simulink model "Boat_Response"  (R2022b)
settings: Solver=VariableStepAuto  StartTime=0.0  StopTime=20  RelTol=0.1
model workspace (MAT data in the model file):
  Air_Kinematic_Viscosity = 1.48e-05
  Air_density = 1.225
  Angle_Breakpoints = [-10.5 -10.25 -10 -9.75 -9.5 -9.25 -9 -8.75 -8.5 -8.25 -8 -7.75 -7.5 -7.25 -7 -6.75 -6.5 -6.25 -6 -5.75 -5.5 -5.25 -5 -4.75 -4.5 -4.25 -4 -3.75 -3.5 -3.25 -3 -2.75 -2.5 -2.25 -2 -1.75 -1.5 -1.25 -1 -0.75 -0.5 -0.25 0 0.25 0.5 0.75 1 1.25 1.5 1.75 2 2.25 2.5 2.75 3 3.25 3.5 3.75 4 4.25 4.5 4.75 5 5.25 5.5 5.75 6 6.25 6.5 6.75 7 7.25 7.5 7.75 8 8.25 8.5 8.75 9 9.25 9.5 9.75 10 10.25 10.5]
  Boat_Slosh_Damping = 1500
  Keel_Area = 1
  Keel_Bulb_COG = 1.3
  Keel_Bulb_Mass = 70
  Keel_Chord = 0.7
  Keel_Fin_COG = 0.8
  Keel_Fin_COP = 0.7
  Keel_Fin_Mass = 8
  M_per_s_to_knots = 1.944
  NACA_0018_Drag_LU = [0.10841 0.10247 0.08947 0.06466 0.05594 0.05095 0.05074 0.04743 0.04673 0.04411 0.04386 0.04172 ... (425 elements, 85x5)]
  NACA_0018_Lift_LU = [-0.4876 -0.5001 -0.5715 -0.7409 -0.8387 -0.8938 -0.8627 -0.8928 -0.8721 -0.8918 -0.8647 -0.8747 ... (425 elements, 85x5)]
  Resistance_Curve = [0; 0.03; 0.11; 0.23; 0.39; 0.58; 0.85; 1.14; 1.49; 1.88; 2.53; 2.87; 3.31; 4.43; 6.4; 6.73; 6.99; 7.38; 13.49; 23.01; 22.15; 20.72; 36.03; 62.97; 86.69; 98.27; 97.94; 90.93; 82.95; 77.95; 77.69; 82.27; 90.87; 102.29; 115.35; 129.07; 142.7; 155.72; 167.84; 178.9; 188.84]
  Resistance_Curve_Velocity_BreakPoints = [0; 0.125; 0.25; 0.375; 0.5; 0.625; 0.75; 0.875; 1; 1.125; 1.25; 1.375; 1.5; 1.625; 1.75; 1.875; 2; 2.125; 2.25; 2.375; 2.5; 2.625; 2.75; 2.875; 3; 3.125; 3.25; 3.375; 3.5; 3.625; 3.75; 3.875; 4; 4.125; 4.25; 4.375; 4.5; 4.625; 4.75; 4.875; 5]
  Reynolds_Breakpoints = [50000 100000 200000 500000 1000000]
  Sail_Area = 2
  Sail_Best_Angles = [5.75 6.75 7 9.25 10]
  Sail_COG = 1.35
  Sail_COP = 1.5
  Sail_Chord = 1.3
  Sail_Mass = 32
  Sig = Simulink.Signal
  Sig.DataType = 'auto'
  Sig.Dimensions = -1
  Sig.DimensionsMode = 'auto'
  Sig.Complexity = 'auto'
  Sig.SampleTime = -1
  Sig.SamplingMode = 'auto'
  Total_MMOI = 200
  Total_Mass = 250
  Water_Density = 997
  Water_Kinematic_Viscosity = 1.3e-06
libraries: simulink_extras x13, vrlib x1, SignalEditorBlockLib x1
settings Model: Creator=ewanb  LastModifiedBy=ewanb
settings SolverCC: ZeroCrossAlgorithm=Adaptive
settings DebuggingCC: IgnoredZcDiagnostic=none

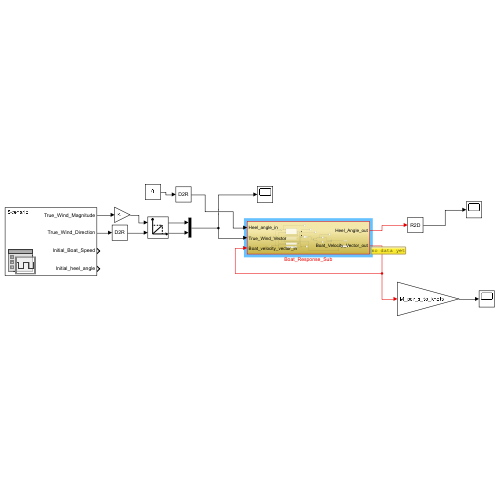
[thumbnail: Simulink's stored preview of the top-level diagram]
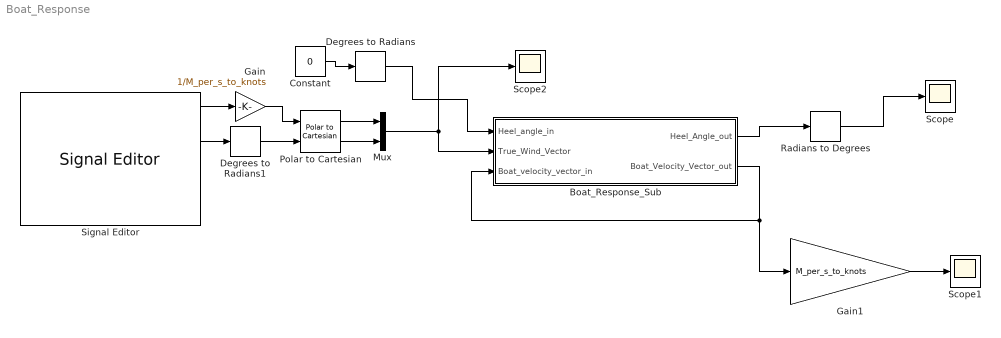
== system Boat_Response ==
  Boat_Response_Sub : Subsystem
  Constant : Constant  Value=0
  Degrees to Radians : simulink_extras/Transformations/Degrees to Radians
  Degrees to Radians1 : simulink_extras/Transformations/Degrees to Radians
  Gain : Gain  Gain=1/M_per_s_to_knots
  Gain1 : Gain  Gain=M_per_s_to_knots
  Mux : Mux  Inputs=2
  Polar to Cartesian : simulink_extras/Transformations/Polar to Cartesian
  Radians to Degrees : simulink_extras/Transformations/Radians to Degrees
  Scope : Scope
  Scope1 : Scope
  Scope2 : Scope
  Signal Editor : SignalEditorBlockLib/Signal Editor  FileName=10knts_Beam_Reach.mat  ActiveScenario=Scenario  ActiveSignal=True_Wind_Magnitude  IsBus=off  OutputBusObjectStr=Bus: BusObject  SampleTime=0  Interpolate=off  ZeroCross=off  OutputAfterFinalValue=Setting to zero  Unit=inherit  PreserveSignalName=on
  wires:
  Polar to Cartesian/1 -> Mux/1
  Mux/1 -> Boat_Response_Sub/2(True_Wind_Vector), Scope2/1
  Polar to Cartesian/2 -> Mux/2
  Radians to Degrees/1 -> Scope/1
  Boat_Response_Sub/1(Heel_Angle_out) -> Radians to Degrees/1
  Boat_Response_Sub/2(Boat_Velocity_Vector_out) -> Gain1/1, Boat_Response_Sub/3(Boat_velocity_vector_in)
  Degrees to Radians1/1 -> Polar to Cartesian/2
  Signal Editor/2 -> Degrees to Radians1/1
  Degrees to Radians/1 -> Boat_Response_Sub/1(Heel_angle_in)
  Constant/1 -> Degrees to Radians/1
  Gain/1 -> Polar to Cartesian/1
  Signal Editor/1 -> Gain/1
  Gain1/1 -> Scope1/1

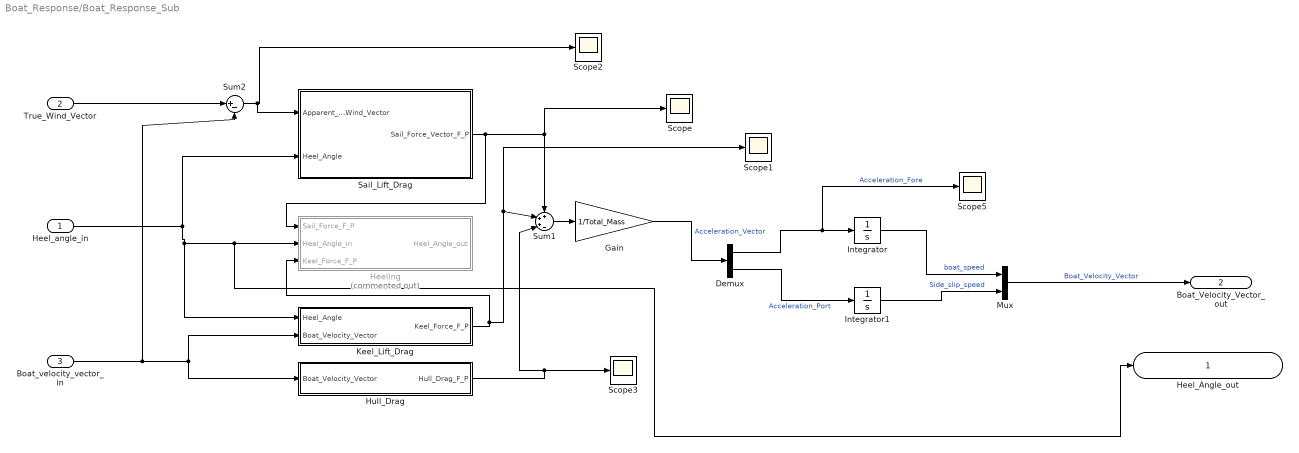
== system Boat_Response/Boat_Response_Sub ==
  Heel_angle_in : Inport
  True_Wind_Vector : Inport  Port=2
  Boat_velocity_vector_in : Inport  Port=3
  Demux : Demux  Outputs=2
  Gain : Gain  Gain=1/Total_Mass
  Heeling : Subsystem  Commented=on
  Hull_Drag : Subsystem
  Integrator : Integrator
  Integrator1 : Integrator
  Keel_Lift_Drag : Subsystem
  Mux : Mux  Inputs=2
  Sail_Lift_Drag : Subsystem
  Scope{,1..3,5} (5 alike) : Scope
  Sum1 : Sum  Inputs=+++-
  Sum2 : Sum  Inputs=|+-
  Heel_Angle_out : Outport
  Boat_Velocity_Vector_out : Outport  Port=2
  wires:
  Mux/1 -> Boat_Velocity_Vector_out/1  "Boat_Velocity_Vector"
  Sum1/1 -> Gain/1
  Boat_velocity_vector_in/1 -> Hull_Drag/1(Boat_Velocity_Vector), Keel_Lift_Drag/2(Boat_Velocity_Vector), Sum2/2
  Keel_Lift_Drag/1(Keel_Force_F_P) -> Heeling/3(Keel_Force_F_P), Sum1/2, Scope1/1
  Demux/1 -> Scope5/1, Integrator/1  "Acceleration_Fore"
  Sum2/1 -> Sail_Lift_Drag/1(Apparent_Wind_Vector), Scope2/1
  Demux/2 -> Integrator1/1  "Acceleration_Port"
  Integrator/1 -> Mux/1  "boat_speed"
  Integrator1/1 -> Mux/2  "Side_slip_speed"
  Gain/1 -> Demux/1  "Acceleration_Vector"
  Sail_Lift_Drag/1(Sail_Force_Vector_F_P) -> Heeling/1(Sail_Force_F_P), Scope/1, Sum1/1
  True_Wind_Vector/1 -> Sum2/1
  Hull_Drag/1(Hull_Drag_F_P) -> Scope3/1, Sum1/3
  Heel_angle_in/1 -> Sail_Lift_Drag/2(Heel_Angle), Keel_Lift_Drag/1(Heel_Angle), Heel_Angle_out/1, Heeling/2(Heel_Angle_in)

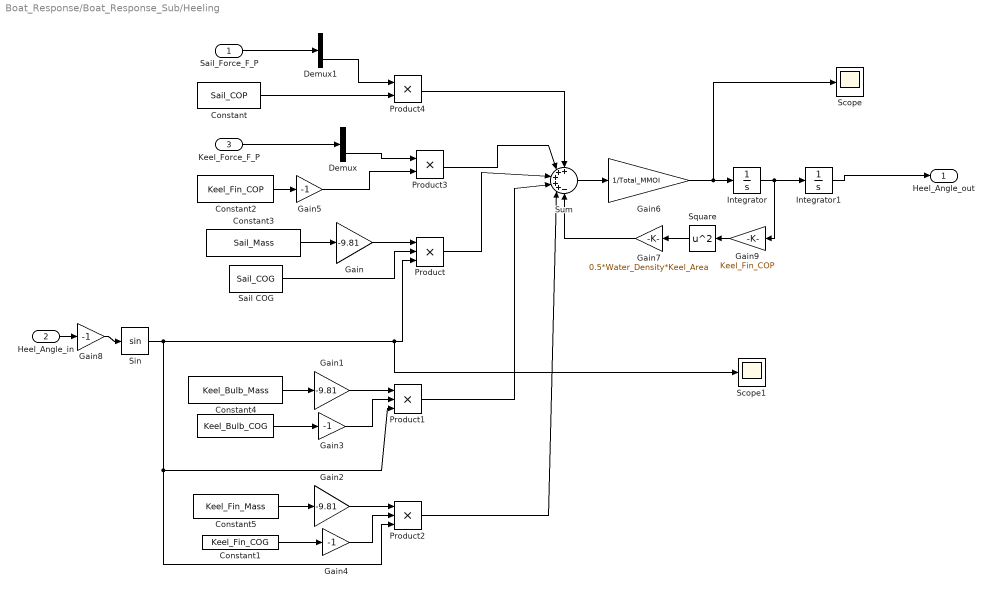
== system Boat_Response/Boat_Response_Sub/Heeling ==
  Sail_Force_F_P : Inport
  Heel_Angle_in : Inport  Port=2
  Keel_Force_F_P : Inport  Port=3
  " " : Constant  Value=Keel_Bulb_COG
  Constant : Constant  Value=Sail_COP
  Constant1 : Constant  Value=Keel_Fin_COG
  Constant2 : Constant  Value=Keel_Fin_COP
  Constant3 : Constant  Value=Sail_Mass
  Constant4 : Constant  Value=Keel_Bulb_Mass
  Constant5 : Constant  Value=Keel_Fin_Mass
  Demux : Demux  Outputs=2
  Demux1 : Demux  Outputs=2
  Gain : Gain  Gain=-9.81
  Gain1 : Gain  Gain=-9.81
  Gain2 : Gain  Gain=-9.81
  Gain{3..5,8} (4 alike) : Gain  Gain=-1
  Gain6 : Gain  Gain=1/Total_MMOI
  Gain7 : Gain  Gain=0.5*Water_Density*Keel_Area
  Gain9 : Gain  Gain=Keel_Fin_COP
  Integrator : Integrator
  Integrator1 : Integrator
  Product : Product  Inputs=3
  Product1 : Product  Inputs=3
  Product2 : Product  Inputs=3
  Product3 : Product
  Product4 : Product
  Sail COG : Constant  Value=Sail_COG
  Scope : Scope
  Scope1 : Scope
  Sin : Trigonometry
  Square : Math  Operator=square
  Sum : Sum  Inputs=+++++-
  Heel_Angle_out : Outport
  wires:
  Constant3/1 -> Gain/1
  Constant4/1 -> Gain1/1
  Constant5/1 -> Gain2/1
  Gain/1 -> Product/1
  Sail COG/1 -> Product/2
  Gain1/1 -> Product1/1
  Gain2/1 -> Product2/1
  Sin/1 -> Product1/3, Product2/3, Scope1/1, Product/3
  " "/1 -> Gain3/1
  Gain3/1 -> Product1/2
  Constant1/1 -> Gain4/1
  Gain4/1 -> Product2/2
  Constant2/1 -> Gain5/1
  Keel_Force_F_P/1 -> Demux/1
  Demux/2 -> Product3/1
  Gain5/1 -> Product3/2
  Sail_Force_F_P/1 -> Demux1/1
  Constant/1 -> Product4/2
  Demux1/2 -> Product4/1
  Product4/1 -> Sum/1
  Product3/1 -> Sum/2
  Product/1 -> Sum/3
  Product1/1 -> Sum/4
  Product2/1 -> Sum/5
  Sum/1 -> Gain6/1
  Integrator/1 -> Gain9/1, Integrator1/1
  Integrator1/1 -> Heel_Angle_out/1
  Gain6/1 -> Scope/1, Integrator/1
  Gain7/1 -> Sum/6
  Heel_Angle_in/1 -> Gain8/1
  Gain8/1 -> Sin/1
  Gain9/1 -> Square/1
  Square/1 -> Gain7/1

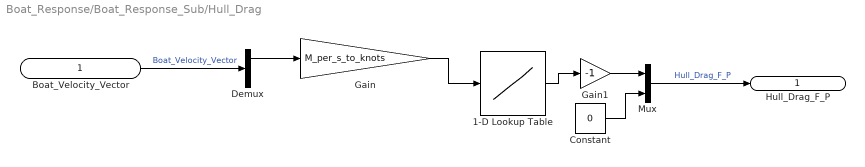
== system Boat_Response/Boat_Response_Sub/Hull_Drag ==
  Boat_Velocity_Vector : Inport
  1-D Lookup Table : Lookup_n-D  NumberOfTableDimensions=1  BreakpointsForDimension1=Resistance_Curve_Velocity_BreakPoints  Table=Resistance_Curve  ExtrapMethod=Clip  UseLastTableValue=on  InternalRulePriority=Speed  RndMeth=Simplest
  Constant : Constant  Value=0
  Demux : Demux  Outputs=2
  Gain : Gain  Gain=M_per_s_to_knots
  Gain1 : Gain  Gain=-1
  Mux : Mux  Inputs=2
  Hull_Drag_F_P : Outport
  wires:
  Gain/1 -> 1-D Lookup Table/1
  Mux/1 -> Hull_Drag_F_P/1  "Hull_Drag_F_P"
  Constant/1 -> Mux/2
  1-D Lookup Table/1 -> Gain1/1
  Gain1/1 -> Mux/1
  Demux/1 -> Gain/1
  Boat_Velocity_Vector/1 -> Demux/1  "Boat_Velocity_Vector"

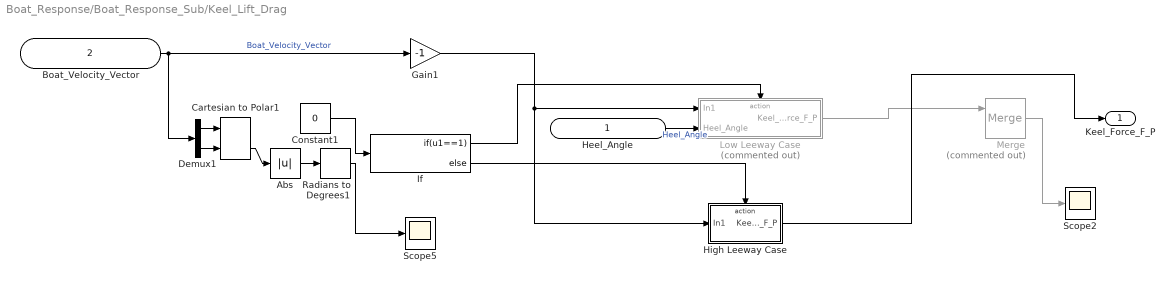
== system Boat_Response/Boat_Response_Sub/Keel_Lift_Drag ==
  Heel_Angle : Inport
  Boat_Velocity_Vector : Inport  Port=2
  Abs : Abs  SaturateOnIntegerOverflow=off
  Cartesian to Polar1 : simulink_extras/Transformations/Cartesian to Polar
  Constant1 : Constant  Value=0
  Demux1 : Demux  Outputs=2
  Gain1 : Gain  Gain=-1
  High Leeway Case : Subsystem  TreatAsAtomicUnit=on
  If : If  IfExpression=u1==1
  Low Leeway Case : Subsystem  Commented=on  TreatAsAtomicUnit=on
  Merge : Merge  Commented=on
  Radians to Degrees1 : simulink_extras/Transformations/Radians to Degrees
  Scope2 : Scope
  Scope5 : Scope
  Keel_Force_F_P : Outport
  wires:
  Boat_Velocity_Vector/1 -> Gain1/1, Demux1/1  "Boat_Velocity_Vector"
  Gain1/1 -> Low Leeway Case/1(In1), High Leeway Case/1(In1)
  Heel_Angle/1 -> Low Leeway Case/2(Heel_Angle)  "Heel_Angle"
  Demux1/1 -> Cartesian to Polar1/1
  Demux1/2 -> Cartesian to Polar1/2
  Cartesian to Polar1/2 -> Abs/1
  Abs/1 -> Radians to Degrees1/1
  Radians to Degrees1/1 -> Scope5/1
  If/1 -> Low Leeway Case/Action
  Low Leeway Case/1(Keel_Force_F_P) -> Merge/1
  Merge/1 -> Scope2/1
  High Leeway Case/1(Keel_Force_F_P) -> Keel_Force_F_P/1
  If/2 -> High Leeway Case/Action
  Constant1/1 -> If/1

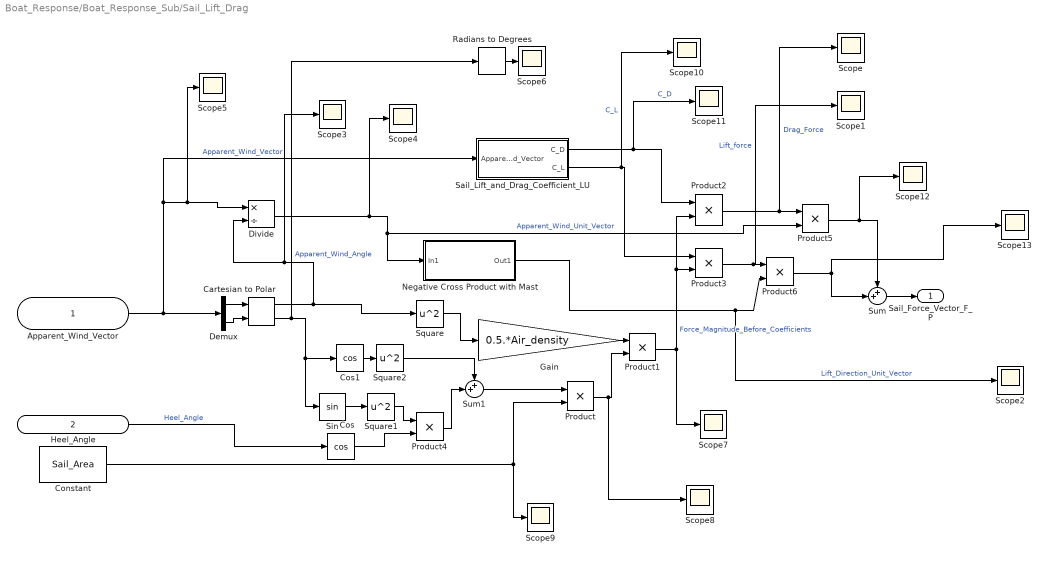
== system Boat_Response/Boat_Response_Sub/Sail_Lift_Drag ==
  Apparent_Wind_Vector : Inport
  Heel_Angle : Inport  Port=2
  Cartesian to Polar : simulink_extras/Transformations/Cartesian to Polar
  Constant : Constant  Value=Sail_Area
  Cos : Trigonometry  Operator=cos
  Cos1 : Trigonometry  Operator=cos
  Demux : Demux  Outputs=2
  Divide : Product  Inputs=*/
  Gain : Gain  Gain=0.5.*Air_density
  Negative Cross Product with Mast : Subsystem
  Product{,1..6} (7 alike) : Product
  Radians to Degrees : simulink_extras/Transformations/Radians to Degrees
  Sail_Lift_and_Drag_Coefficient_LU : Subsystem
  Scope{,1..13} (14 alike) : Scope
  Sin : Trigonometry
  Square : Math  Operator=square
  Square1 : Math  Operator=square
  Square2 : Math  Operator=square
  Sum : Sum  Inputs=++|
  Sum1 : Sum  Inputs=++|
  Sail_Force_Vector_F_P : Outport
  wires:
  Apparent_Wind_Vector/1 -> Sail_Lift_and_Drag_Coefficient_LU/1(Apparent_Wind_Vector), Scope5/1, Divide/1, Demux/1  "Apparent_Wind_Vector"
  Demux/1 -> Cartesian to Polar/1
  Demux/2 -> Cartesian to Polar/2
  Cartesian to Polar/1 -> Scope3/1, Divide/2, Square/1
  Heel_Angle/1 -> Cos/1  "Heel_Angle"
  Cartesian to Polar/2 -> Radians to Degrees/1, Cos1/1, Sin/1  "Apparent_Wind_Angle"
  Square/1 -> Gain/1
  Product/1 -> Scope8/1, Product1/2
  Gain/1 -> Product1/1
  Divide/1 -> Scope4/1, Product5/2, Negative Cross Product with Mast/1(In1)  "Apparent_Wind_Unit_Vector"
  Sail_Lift_and_Drag_Coefficient_LU/2(C_L) -> Scope10/1, Product3/1  "C_L"
  Sail_Lift_and_Drag_Coefficient_LU/1(C_D) -> Scope11/1, Product2/1  "C_D"
  Sum/1 -> Sail_Force_Vector_F_P/1
  Cos/1 -> Product4/2
  Product4/1 -> Sum1/2
  Constant/1 -> Product/2, Scope9/1
  Sum1/1 -> Product/1
  Product1/1 -> Product2/2, Product3/2, Scope7/1  "Force_Magnitude_Before_Coefficients"
  Product2/1 -> Scope/1, Product5/1  "Drag_Force"
  Negative Cross Product with Mast/1(Out1) -> Scope2/1, Product6/2  "Lift_Direction_Unit_Vector"
  Product3/1 -> Scope1/1, Product6/1  "Lift_force"
  Product6/1 -> Sum/2, Scope13/1
  Product5/1 -> Scope12/1, Sum/1
  Sin/1 -> Square1/1
  Square1/1 -> Product4/1
  Cos1/1 -> Square2/1
  Square2/1 -> Sum1/1
  Radians to Degrees/1 -> Scope6/1

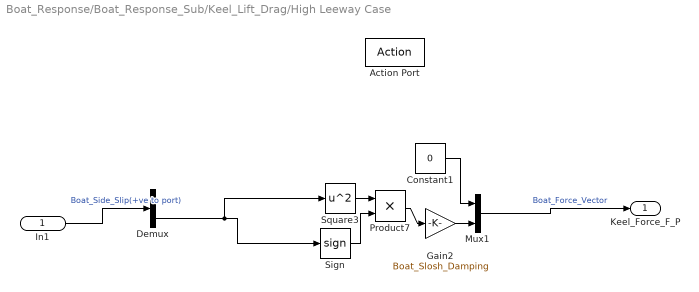
== system Boat_Response/Boat_Response_Sub/Keel_Lift_Drag/High Leeway Case ==
  In1 : Inport
  Action Port : ActionPort  ActionPortLabel=else
  Constant1 : Constant  Value=0
  Demux : Demux  Outputs=2
  Gain2 : Gain  Gain=Boat_Slosh_Damping
  Mux1 : Mux  Inputs=2
  Product7 : Product
  Sign : Signum
  Square3 : Math  Operator=square
  Keel_Force_F_P : Outport
  wires:
  Square3/1 -> Product7/1
  Sign/1 -> Product7/2
  Constant1/1 -> Mux1/1
  Gain2/1 -> Mux1/2
  Product7/1 -> Gain2/1
  Mux1/1 -> Keel_Force_F_P/1  "Boat_Force_Vector"
  In1/1 -> Demux/1  "Boat_Side_Slip(+ve to port)"
  Demux/2 -> Square3/1, Sign/1

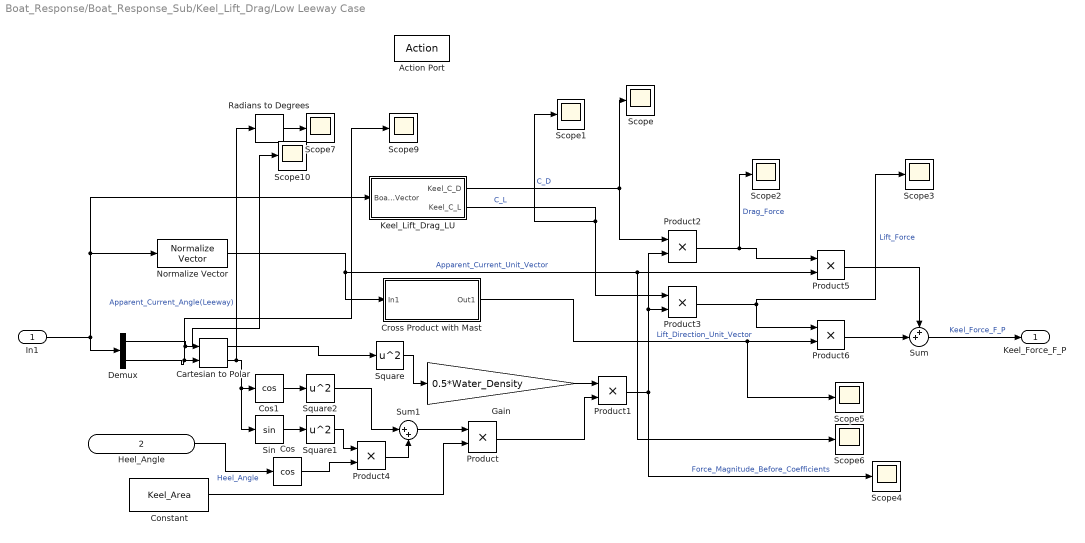
== system Boat_Response/Boat_Response_Sub/Keel_Lift_Drag/Low Leeway Case ==
  In1 : Inport
  Heel_Angle : Inport  Port=2
  Action Port : ActionPort  ActionPortLabel=if(u1 < 5)
  Cartesian to Polar : simulink_extras/Transformations/Cartesian to Polar
  Constant : Constant  Value=Keel_Area
  Cos : Trigonometry  Operator=cos
  Cos1 : Trigonometry  Operator=cos
  Cross Product with Mast : Subsystem
  Demux : Demux  Outputs=2
  Gain : Gain  Gain=0.5*Water_Density
  Keel_Lift_Drag_LU : Subsystem
  Normalize Vector : vrlib/Utilities/Normalize Vector  maxzero=0
  Product{,1..6} (7 alike) : Product
  Radians to Degrees : simulink_extras/Transformations/Radians to Degrees
  Scope{,1..7,9..10} (10 alike) : Scope
  Sin : Trigonometry
  Square : Math  Operator=square
  Square1 : Math  Operator=square
  Square2 : Math  Operator=square
  Sum : Sum  Inputs=++|
  Sum1 : Sum  Inputs=|++
  Keel_Force_F_P : Outport
  wires:
  Demux/2 -> Scope9/1, Cartesian to Polar/2
  In1/1 -> Demux/1, Keel_Lift_Drag_LU/1(Boat_Velocity_Vector), Normalize Vector/1
  Product3/1 -> Product6/1, Scope3/1  "Lift_Force"
  Cos/1 -> Product4/2
  Constant/1 -> Product/2
  Cross Product with Mast/1(Out1) -> Scope5/1, Product6/2  "Lift_Direction_Unit_Vector"
  Radians to Degrees/1 -> Scope7/1
  Product2/1 -> Scope2/1, Product5/1  "Drag_Force"
  Product5/1 -> Sum/1
  Square1/1 -> Product4/1
  Sin/1 -> Square1/1
  Product1/1 -> Product2/2, Product3/2, Scope4/1  "Force_Magnitude_Before_Coefficients"
  Cartesian to Polar/1 -> Square/1
  Product6/1 -> Sum/2
  Normalize Vector/1 -> Scope6/1, Product5/2, Cross Product with Mast/1(In1)  "Apparent_Current_Unit_Vector"
  Sum/1 -> Keel_Force_F_P/1  "Keel_Force_F_P"
  Keel_Lift_Drag_LU/2(Keel_C_L) -> Scope1/1, Product3/1  "C_L"
  Keel_Lift_Drag_LU/1(Keel_C_D) -> Scope/1, Product2/1  "C_D"
  Heel_Angle/1 -> Cos/1  "Heel_Angle"
  Product/1 -> Product1/2
  Gain/1 -> Product1/1
  Demux/1 -> Scope10/1, Cartesian to Polar/1
  Cartesian to Polar/2 -> Radians to Degrees/1, Cos1/1, Sin/1  "Apparent_Current_Angle(Leeway)"
  Product4/1 -> Sum1/2
  Cos1/1 -> Square2/1
  Square2/1 -> Sum1/1
  Square/1 -> Gain/1
  Sum1/1 -> Product/1

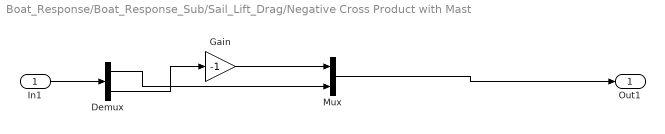
== system Boat_Response/Boat_Response_Sub/Sail_Lift_Drag/Negative Cross Product with Mast ==
  In1 : Inport
  Demux : Demux  Outputs=2
  Gain : Gain  Gain=-1
  Mux : Mux  Inputs=2
  Out1 : Outport
  wires:
  In1/1 -> Demux/1
  Mux/1 -> Out1/1
  Demux/1 -> Mux/2
  Demux/2 -> Gain/1
  Gain/1 -> Mux/1

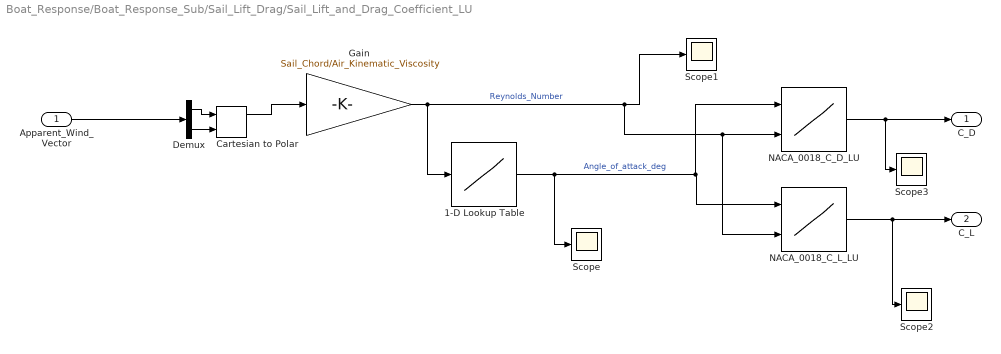
== system Boat_Response/Boat_Response_Sub/Sail_Lift_Drag/Sail_Lift_and_Drag_Coefficient_LU ==
  Apparent_Wind_Vector : Inport
  1-D Lookup Table : Lookup_n-D  NumberOfTableDimensions=1  BreakpointsForDimension1=Reynolds_Breakpoints  Table=Sail_Best_Angles  InterpMethod=Nearest  InternalRulePriority=Speed  RndMeth=Simplest
  Cartesian to Polar : simulink_extras/Transformations/Cartesian to Polar
  Demux : Demux  Outputs=2
  Gain : Gain  Gain=Sail_Chord/Air_Kinematic_Viscosity
  NACA_0018_C_D_LU : Lookup_n-D  LookupTableObject=''  BreakpointsForDimension1=Angle_Breakpoints  BreakpointsForDimension2=Reynolds_Breakpoints  BreakpointsForDimension1FirstPoint=10  BreakpointsForDimension2FirstPoint=10  BreakpointsForDimension1Spacing=12  BreakpointsForDimension2Spacing=12  IndexSearchMethod=Linear search  Table=NACA_0018_Drag_LU  InterpMethod=Nearest  DiagnosticForOutOfRangeInput=Warning  InternalRulePriority=Speed  RndMeth=Simplest
      settings: InputPortMap=u0,u1
  NACA_0018_C_L_LU : Lookup_n-D  LookupTableObject=''  BreakpointsForDimension1=Angle_Breakpoints  BreakpointsForDimension2=Reynolds_Breakpoints  BreakpointsForDimension1FirstPoint=10  BreakpointsForDimension2FirstPoint=10  BreakpointsForDimension1Spacing=12  BreakpointsForDimension2Spacing=12  Table=NACA_0018_Lift_LU  InterpMethod=Nearest  DiagnosticForOutOfRangeInput=Warning  InternalRulePriority=Speed  RndMeth=Simplest
      settings: InputPortMap=u0,u1
  Scope{,1..3} (4 alike) : Scope
  C_D : Outport
  C_L : Outport  Port=2
  wires:
  NACA_0018_C_D_LU/1 -> Scope3/1, C_D/1
  NACA_0018_C_L_LU/1 -> Scope2/1, C_L/1
  Cartesian to Polar/1 -> Gain/1
  Demux/2 -> Cartesian to Polar/2
  1-D Lookup Table/1 -> Scope/1, NACA_0018_C_D_LU/1, NACA_0018_C_L_LU/1  "Angle_of_attack_deg"
  Gain/1 -> NACA_0018_C_L_LU/2, NACA_0018_C_D_LU/2, Scope1/1, 1-D Lookup Table/1  "Reynolds_Number"
  Demux/1 -> Cartesian to Polar/1
  Apparent_Wind_Vector/1 -> Demux/1

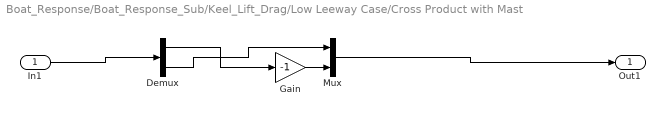
== system Boat_Response/Boat_Response_Sub/Keel_Lift_Drag/Low Leeway Case/Cross Product with Mast ==
  In1 : Inport
  Demux : Demux  Outputs=2
  Gain : Gain  Gain=-1
  Mux : Mux  Inputs=2
  Out1 : Outport
  wires:
  In1/1 -> Demux/1
  Mux/1 -> Out1/1
  Gain/1 -> Mux/2
  Demux/1 -> Gain/1
  Demux/2 -> Mux/1

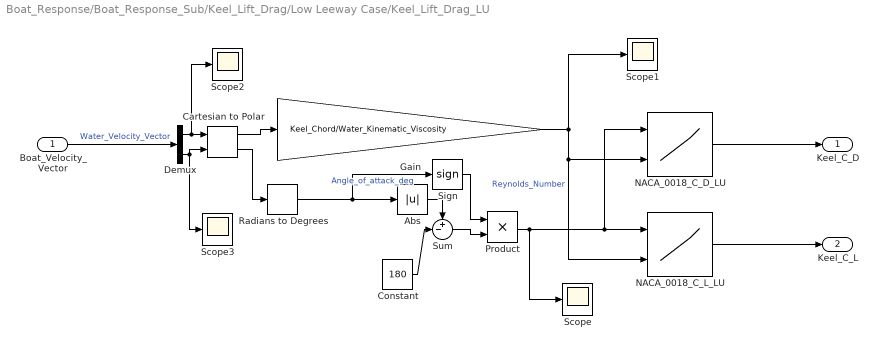
== system Boat_Response/Boat_Response_Sub/Keel_Lift_Drag/Low Leeway Case/Keel_Lift_Drag_LU ==
  Boat_Velocity_Vector : Inport
  Abs : Abs  SaturateOnIntegerOverflow=off
  Cartesian to Polar : simulink_extras/Transformations/Cartesian to Polar
  Constant : Constant  Value=180
  Demux : Demux  Outputs=2
  Gain : Gain  Gain=Keel_Chord/Water_Kinematic_Viscosity
  NACA_0018_C_D_LU : Lookup_n-D  LookupTableObject=''  BreakpointsForDimension1=Angle_Breakpoints  BreakpointsForDimension2=Reynolds_Breakpoints  BreakpointsForDimension1FirstPoint=10  BreakpointsForDimension2FirstPoint=10  BreakpointsForDimension1Spacing=12  BreakpointsForDimension2Spacing=12  IndexSearchMethod=Linear search  Table=NACA_0018_Drag_LU  InterpMethod=Flat  DiagnosticForOutOfRangeInput=Warning  InternalRulePriority=Speed  RndMeth=Simplest
      settings: InputPortMap=u0,u1
  NACA_0018_C_L_LU : Lookup_n-D  LookupTableObject=''  BreakpointsForDimension1=Angle_Breakpoints  BreakpointsForDimension2=Reynolds_Breakpoints  BreakpointsForDimension1FirstPoint=10  BreakpointsForDimension2FirstPoint=10  BreakpointsForDimension1Spacing=12  BreakpointsForDimension2Spacing=12  IndexSearchMethod=Linear search  Table=NACA_0018_Lift_LU  InterpMethod=Flat  DiagnosticForOutOfRangeInput=Warning  InternalRulePriority=Speed  RndMeth=Simplest
      settings: InputPortMap=u0,u1
  Product : Product
  Radians to Degrees : simulink_extras/Transformations/Radians to Degrees
  Scope{,1..3} (4 alike) : Scope
  Sign : Signum
  Sum : Sum  Inputs=+-|
  Keel_C_D : Outport
  Keel_C_L : Outport  Port=2
  wires:
  Boat_Velocity_Vector/1 -> Demux/1  "Water_Velocity_Vector"
  Demux/1 -> Scope2/1, Cartesian to Polar/1
  Demux/2 -> Scope3/1, Cartesian to Polar/2
  Cartesian to Polar/1 -> Gain/1
  Cartesian to Polar/2 -> Radians to Degrees/1
  Gain/1 -> NACA_0018_C_L_LU/2, NACA_0018_C_D_LU/2, Scope1/1  "Reynolds_Number"
  NACA_0018_C_D_LU/1 -> Keel_C_D/1
  NACA_0018_C_L_LU/1 -> Keel_C_L/1
  Radians to Degrees/1 -> Sign/1, Abs/1  "Angle_of_attack_deg"
  Abs/1 -> Sum/1
  Constant/1 -> Sum/2
  Sum/1 -> Product/2
  Sign/1 -> Product/1
  Product/1 -> Scope/1, NACA_0018_C_D_LU/1, NACA_0018_C_L_LU/1
